simulink library "slQuery_testlibrary"  (Simulink 10.0)
settings: Solver=VariableStepAuto  StartTime=0.0  StopTime=10.0  RelTol=1e-3  EnableMultiTasking=on
libraries: $bdroot x39
settings Model: Creator=FO10C9R  LastModifiedBy=FO10C9R

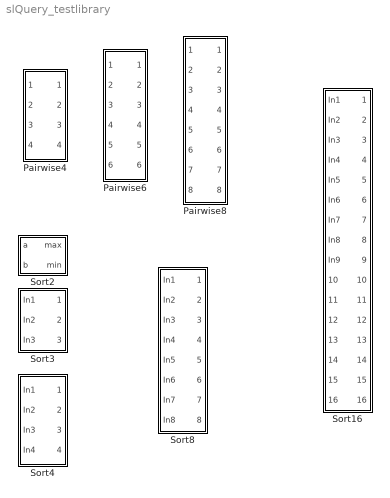
== system slQuery_testlibrary ==
  Pairwise4 : Subsystem
      mask Display: disp(['1-4' 10 '2-3'])
  Pairwise6 : Subsystem
      mask Display: disp(['1-6' 10 '2-5' 10 '3-4'])
  Pairwise8 : Subsystem
      mask Display: disp(['1-8' 10 '2-7' 10 '3-6' 10 '4-5'])
  Sort16 : Subsystem  mask(Sort){}
      mask Display: disp('>O(44)')
  Sort2 : Subsystem  mask(Sort){}
      mask Display: disp('O(1)')
  Sort3 : Subsystem  mask(Sort){}
      mask Display: disp('O(3)')
  Sort4 : Subsystem  mask(Sort){}
      mask Display: disp('O(5)')
  Sort8 : Subsystem  mask(Sort){}
      mask Display: disp('O(19)')

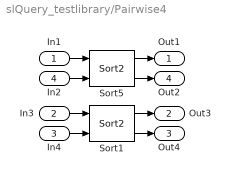
== system slQuery_testlibrary/Pairwise4 ==
  In1 : Inport
  In3 : Inport  Port=2
  In4 : Inport  Port=3
  In2 : Inport  Port=4
  Sort1 : $bdroot/Sort2  SystemSampleTime=-1
  Sort5 : $bdroot/Sort2  SystemSampleTime=-1
  Out1 : Outport
  Out3 : Outport  Port=2
  Out4 : Outport  Port=3
  Out2 : Outport  Port=4
  wires:
  Sort1/2 -> Out4/1
  Sort5/2 -> Out2/1
  In1/1 -> Sort5/1
  Sort1/1 -> Out3/1
  In3/1 -> Sort1/1
  In2/1 -> Sort5/2
  In4/1 -> Sort1/2
  Sort5/1 -> Out1/1

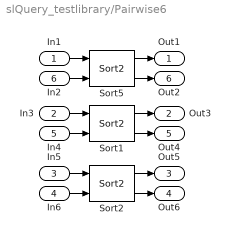
== system slQuery_testlibrary/Pairwise6 ==
  In1 : Inport
  In3 : Inport  Port=2
  In5 : Inport  Port=3
  In6 : Inport  Port=4
  In4 : Inport  Port=5
  In2 : Inport  Port=6
  Sort1 : $bdroot/Sort2  SystemSampleTime=-1
  Sort2 : $bdroot/Sort2  SystemSampleTime=-1
  Sort5 : $bdroot/Sort2  SystemSampleTime=-1
  Out1 : Outport
  Out3 : Outport  Port=2
  Out5 : Outport  Port=3
  Out6 : Outport  Port=4
  Out4 : Outport  Port=5
  Out2 : Outport  Port=6
  wires:
  Sort5/1 -> Out1/1
  In4/1 -> Sort1/2
  In2/1 -> Sort5/2
  In3/1 -> Sort1/1
  Sort1/1 -> Out3/1
  In1/1 -> Sort5/1
  Sort5/2 -> Out2/1
  Sort1/2 -> Out4/1
  In6/1 -> Sort2/2
  In5/1 -> Sort2/1
  Sort2/1 -> Out5/1
  Sort2/2 -> Out6/1

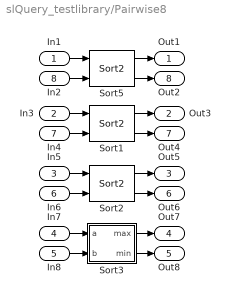
== system slQuery_testlibrary/Pairwise8 ==
  In1 : Inport
  In3 : Inport  Port=2
  In5 : Inport  Port=3
  In7 : Inport  Port=4
  In8 : Inport  Port=5
  In6 : Inport  Port=6
  In4 : Inport  Port=7
  In2 : Inport  Port=8
  Sort1 : $bdroot/Sort2  SystemSampleTime=-1
  Sort2 : $bdroot/Sort2  SystemSampleTime=-1
  Sort3 : Subsystem  mask(Sort){}
      mask Display: disp('O(1)')
  Sort5 : $bdroot/Sort2  SystemSampleTime=-1
  Out1 : Outport
  Out3 : Outport  Port=2
  Out5 : Outport  Port=3
  Out7 : Outport  Port=4
  Out8 : Outport  Port=5
  Out6 : Outport  Port=6
  Out4 : Outport  Port=7
  Out2 : Outport  Port=8
  wires:
  Sort2/2 -> Out6/1
  Sort2/1 -> Out5/1
  In5/1 -> Sort2/1
  In6/1 -> Sort2/2
  Sort1/2 -> Out4/1
  Sort5/2 -> Out2/1
  In1/1 -> Sort5/1
  Sort1/1 -> Out3/1
  In3/1 -> Sort1/1
  In2/1 -> Sort5/2
  In4/1 -> Sort1/2
  Sort5/1 -> Out1/1
  Sort3/2(min) -> Out8/1
  Sort3/1(max) -> Out7/1
  In7/1 -> Sort3/1(a)
  In8/1 -> Sort3/2(b)

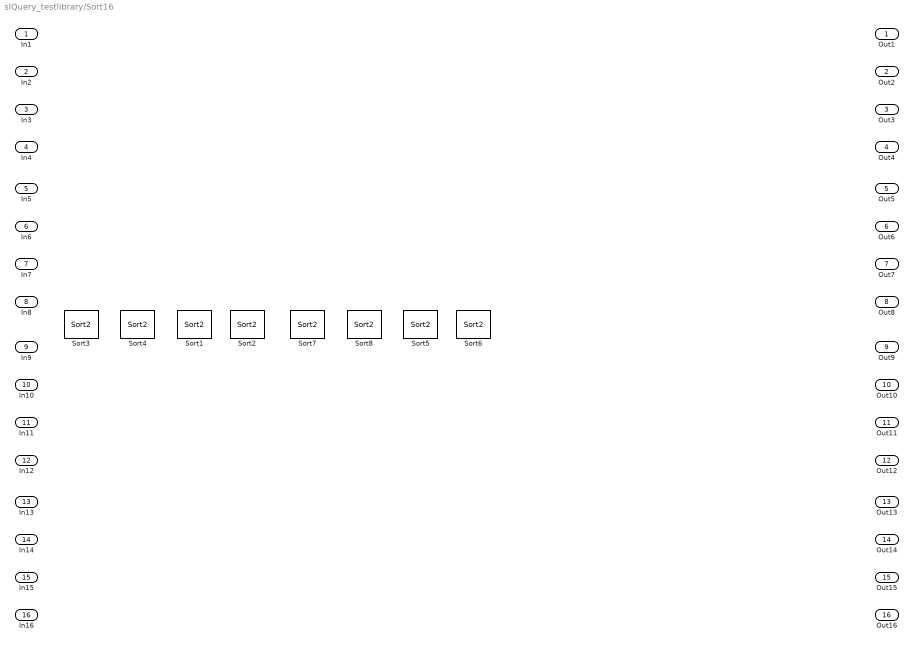
== system slQuery_testlibrary/Sort16 ==
  In1 : Inport
  In2 : Inport  Port=2
  In3 : Inport  Port=3
  In4 : Inport  Port=4
  In5 : Inport  Port=5
  In6 : Inport  Port=6
  In7 : Inport  Port=7
  In8 : Inport  Port=8
  In9 : Inport  Port=9
  In10 : Inport  Port=10
  In11 : Inport  Port=11
  In12 : Inport  Port=12
  In13 : Inport  Port=13
  In14 : Inport  Port=14
  In15 : Inport  Port=15
  In16 : Inport  Port=16
  Sort{1..8} (8 alike) : $bdroot/Sort2  SystemSampleTime=-1
  Out1 : Outport
  Out2 : Outport  Port=2
  Out3 : Outport  Port=3
  Out4 : Outport  Port=4
  Out5 : Outport  Port=5
  Out6 : Outport  Port=6
  Out7 : Outport  Port=7
  Out8 : Outport  Port=8
  Out9 : Outport  Port=9
  Out10 : Outport  Port=10
  Out11 : Outport  Port=11
  Out12 : Outport  Port=12
  Out13 : Outport  Port=13
  Out14 : Outport  Port=14
  Out15 : Outport  Port=15
  Out16 : Outport  Port=16

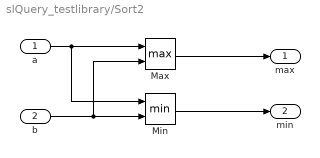
== system slQuery_testlibrary/Sort2 ==
  a : Inport
  b : Inport  Port=2
  Max : MinMax  Function=max  Inputs=2
  Min : MinMax  Inputs=2
  max : Outport
  min : Outport  Port=2
  wires:
  a/1 -> Min/1, Max/1
  b/1 -> Max/2, Min/2
  Min/1 -> min/1
  Max/1 -> max/1

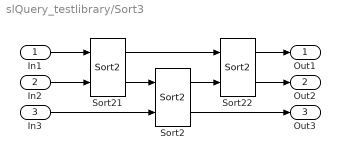
== system slQuery_testlibrary/Sort3 ==
  In1 : Inport
  In2 : Inport  Port=2
  In3 : Inport  Port=3
  Sort2 : $bdroot/Sort2  SystemSampleTime=-1
  Sort21 : $bdroot/Sort2  SystemSampleTime=-1
  Sort22 : $bdroot/Sort2  SystemSampleTime=-1
  Out1 : Outport
  Out2 : Outport  Port=2
  Out3 : Outport  Port=3
  wires:
  In1/1 -> Sort21/1
  In3/1 -> Sort2/2
  In2/1 -> Sort21/2
  Sort2/2 -> Out3/1
  Sort21/2 -> Sort2/1
  Sort2/1 -> Sort22/2
  Sort21/1 -> Sort22/1
  Sort22/1 -> Out1/1
  Sort22/2 -> Out2/1

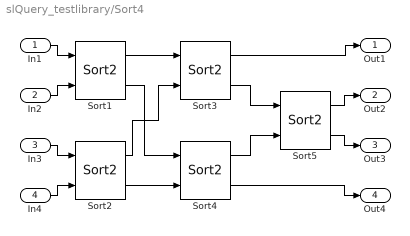
== system slQuery_testlibrary/Sort4 ==
  In1 : Inport
  In2 : Inport  Port=2
  In3 : Inport  Port=3
  In4 : Inport  Port=4
  Sort{1..5} (5 alike) : $bdroot/Sort2  SystemSampleTime=-1
  Out1 : Outport
  Out2 : Outport  Port=2
  Out3 : Outport  Port=3
  Out4 : Outport  Port=4
  wires:
  In1/1 -> Sort1/1
  In2/1 -> Sort1/2
  In3/1 -> Sort2/1
  In4/1 -> Sort2/2
  Sort1/1 -> Sort3/1
  Sort2/1 -> Sort3/2
  Sort3/1 -> Out1/1
  Sort4/2 -> Out4/1
  Sort2/2 -> Sort4/2
  Sort1/2 -> Sort4/1
  Sort5/1 -> Out2/1
  Sort5/2 -> Out3/1
  Sort3/2 -> Sort5/1
  Sort4/1 -> Sort5/2

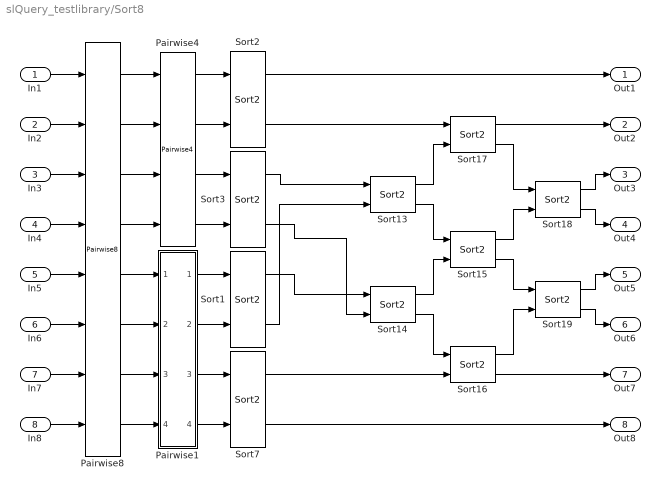
== system slQuery_testlibrary/Sort8 ==
  In1 : Inport
  In2 : Inport  Port=2
  In3 : Inport  Port=3
  In4 : Inport  Port=4
  In5 : Inport  Port=5
  In6 : Inport  Port=6
  In7 : Inport  Port=7
  In8 : Inport  Port=8
  Pairwise1 : Subsystem
      mask Display: disp(['1-4' 10 '2-3'])
  Pairwise4 : $bdroot/Pairwise4  SystemSampleTime=-1
  Pairwise8 : $bdroot/Pairwise8  SystemSampleTime=-1
  Sort{1..3,7,13..19} (11 alike) : $bdroot/Sort2  SystemSampleTime=-1
  Out1 : Outport
  Out2 : Outport  Port=2
  Out3 : Outport  Port=3
  Out4 : Outport  Port=4
  Out5 : Outport  Port=5
  Out6 : Outport  Port=6
  Out7 : Outport  Port=7
  Out8 : Outport  Port=8
  wires:
  Sort3/1 -> Sort13/1
  Sort1/2 -> Sort13/2
  Sort3/2 -> Sort14/2
  Sort1/1 -> Sort14/1
  Sort2/1 -> Out1/1
  Sort7/2 -> Out8/1
  Sort2/2 -> Sort17/1
  Sort13/1 -> Sort17/2
  Sort17/1 -> Out2/1
  Sort17/2 -> Sort18/1
  Sort18/1 -> Out3/1
  Sort13/2 -> Sort15/1
  Sort15/1 -> Sort18/2
  Sort14/1 -> Sort15/2
  Sort15/2 -> Sort19/1
  Sort16/1 -> Sort19/2
  Sort14/2 -> Sort16/1
  Sort7/1 -> Sort16/2
  Sort16/2 -> Out7/1
  Sort19/2 -> Out6/1
  Sort19/1 -> Out5/1
  Sort18/2 -> Out4/1
  In1/1 -> Pairwise8/1
  In2/1 -> Pairwise8/2
  In3/1 -> Pairwise8/3
  In4/1 -> Pairwise8/4
  In5/1 -> Pairwise8/5
  In6/1 -> Pairwise8/6
  In7/1 -> Pairwise8/7
  In8/1 -> Pairwise8/8
  Pairwise8/1 -> Pairwise4/1
  Pairwise8/2 -> Pairwise4/2
  Pairwise8/3 -> Pairwise4/3
  Pairwise8/4 -> Pairwise4/4
  Pairwise8/5 -> Pairwise1/1(In1)
  Pairwise8/6 -> Pairwise1/2(In3)
  Pairwise8/7 -> Pairwise1/3(In4)
  Pairwise8/8 -> Pairwise1/4(In2)
  Pairwise1/4(Out2) -> Sort7/2
  Pairwise1/3(Out4) -> Sort7/1
  Pairwise1/1(Out1) -> Sort1/1
  Pairwise1/2(Out3) -> Sort1/2
  Pairwise4/3 -> Sort3/1
  Pairwise4/4 -> Sort3/2
  Pairwise4/1 -> Sort2/1
  Pairwise4/2 -> Sort2/2

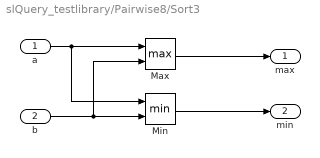
== system slQuery_testlibrary/Pairwise8/Sort3 ==
  a : Inport
  b : Inport  Port=2
  Max : MinMax  Function=max  Inputs=2
  Min : MinMax  Inputs=2
  max : Outport
  min : Outport  Port=2
  wires:
  Max/1 -> max/1
  Min/1 -> min/1
  b/1 -> Min/2, Max/2
  a/1 -> Max/1, Min/1

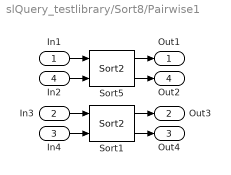
== system slQuery_testlibrary/Sort8/Pairwise1 ==
  In1 : Inport
  In3 : Inport  Port=2
  In4 : Inport  Port=3
  In2 : Inport  Port=4
  Sort1 : $bdroot/Sort2  SystemSampleTime=-1
  Sort5 : $bdroot/Sort2  SystemSampleTime=-1
  Out1 : Outport
  Out3 : Outport  Port=2
  Out4 : Outport  Port=3
  Out2 : Outport  Port=4
  wires:
  Sort5/1 -> Out1/1
  In4/1 -> Sort1/2
  In2/1 -> Sort5/2
  In3/1 -> Sort1/1
  Sort1/1 -> Out3/1
  In1/1 -> Sort5/1
  Sort5/2 -> Out2/1
  Sort1/2 -> Out4/1
